simulink model "Quadrotor_Controller"  (R2019a)
settings: Solver=ode14x  StartTime=0.0  StopTime=10  FixedStep=1/100  RelTol=1e-3  EnableMultiTasking=on
undefined symbols (not defined in the file): Ap, cd, dfod, DiscIntNeverNeededParam, ioKd, ioKi, ioKp, Kd, Kp, kt, L, Newton, Pitch_0, Raphson, rho, Roll_0, Rp, X, Y, Z
libraries: sm_lib x122, fl_ps_legacy_lib x41, fl_lib x28, nesl_utility x14, sharedtransform x12, simulink x5, Electrical_Library x4, Mechanical_Library x4
(part 2 of 5)

== system Quadrotor_Controller/Controller/FOPI- GNCC IRID ==
  note: gam=-0.9693;
      | Ts=0.01;
      | dfod=irid_fod(gam,Ts,5);
  note: FOPI GNCC IRID
  In1 : Inport
  Discrete Transfer Fcn : DiscreteTransferFcn  Numerator=[0.0101201839324044,-0.0228427827690589,0.0162967440497079,-0.00320636053105791,-0.000423005899049262,8.95094110425754e-05]  Denominator=[1,-3.37446144143197,4.28685637101180,-2.49589501448942,0.632511381183536,-0.0490106070515154]
  Fractional DD : Subsystem  Commented=through  mask{gam=0.9693, ww=[1e-4,1e4], n=6, kF1=on, kF=Oustaloup filter, Ts=0.01}
      mask prompts: gam "Derivative order gamma"; ww "Frequency range [wb,wh]"; n "Apprixmation order"; kF1 "Is a low-pass filter required?"; kF "Filter type"; Ts "Sampling period"
      mask init: same as Quadrotor_Controller/Controller/FOPD/Fractional DD
      mask TypeOptions kF: Oustaloup filter | Modified Oustaloup filter | Matsuda-Fujii filter
      mask Display: disp(str)
  Saturation1 : Saturate  Commented=through  UpperLimit=2e3  LowerLimit=-2e3
  Saturation2 : Saturate  Commented=through  UpperLimit=100  LowerLimit=-100
  Sum : Sum
  k_i : Gain  Gain=0.1631
  k_p : Gain  Gain=9.9498
  Out1 : Outport
  wires:
  Fractional DD/1(Out1) -> Discrete Transfer Fcn/1  "DD_out"
  k_i/1 -> Fractional DD/1(In1)  "DD_input"
  In1/1 -> Sum/1, k_i/1  "P"
  Sum/1 -> k_p/1
  k_p/1 -> Saturation1/1
  Saturation1/1 -> Out1/1
  Saturation2/1 -> Sum/2  "D"
  Discrete Transfer Fcn/1 -> Saturation2/1

== system Quadrotor_Controller/Controller/FOPID ==
  note: FOPID controller
  In1 : Inport
  Fractional DD : Subsystem  mask{gam=0, ww=[1e-4,1e4], n=6, kF1=on, kF=Oustaloup filter, Ts=0.01}
      mask prompts: gam "Derivative order gamma"; ww "Frequency range [wb,wh]"; n "Apprixmation order"; kF1 "Is a low-pass filter required?"; kF "Filter type"; Ts "Sampling period"
      mask init: same as Quadrotor_Controller/Controller/FOPD/Fractional DD
      mask TypeOptions kF: Oustaloup filter | Modified Oustaloup filter | Matsuda-Fujii filter
      mask Display: disp(str)
  Fractional DD1 : Subsystem  mask{gam=1.5, ww=[1e-4,1e4], n=6, kF1=on, kF=Oustaloup filter, Ts=0.01}
      mask prompts: gam "Derivative order gamma"; ww "Frequency range [wb,wh]"; n "Apprixmation order"; kF1 "Is a low-pass filter required?"; kF "Filter type"; Ts "Sampling period"
      mask init: same as Quadrotor_Controller/Controller/FOPD/Fractional DD
      mask TypeOptions kF: Oustaloup filter | Modified Oustaloup filter | Matsuda-Fujii filter
      mask Display: disp(str)
  Gain1 : Gain  Gain=0
  Gain2 : Gain  Gain=2.6
  Gain3 : Gain  Gain=1.631
  Saturation1 : Saturate  UpperLimit=2e3  LowerLimit=-2e3
  Saturation2 : Saturate  UpperLimit=100  LowerLimit=-100
  Saturation3 : Saturate  UpperLimit=100  LowerLimit=-100
  Sum : Sum  Inputs=+++
  Out1 : Outport
  wires:
  Fractional DD/1(Out1) -> Saturation2/1  "DD_out"
  Gain1/1 -> Fractional DD/1(In1)  "DD_input"
  In1/1 -> Gain2/1, Gain3/1, Gain1/1  "P"
  Sum/1 -> Saturation1/1
  Saturation1/1 -> Out1/1
  Saturation2/1 -> Sum/2  "D"
  Gain2/1 -> Sum/1  "DD_input"
  Gain3/1 -> Fractional DD1/1(In1)  "DD_input"
  Fractional DD1/1(Out1) -> Saturation3/1  "DD_out"
  Saturation3/1 -> Sum/3  "D"

== system Quadrotor_Controller/Controller/FOPID NPM IRID with correct plant ==
  note: FOPID controller
  In1 : Inport
  Discrete Transfer Fcn : DiscreteTransferFcn  Numerator=[1,-3.16336631308587,3.71959536925849,-1.96568707629962,0.436885459917815,-0.0273811687803932]  Denominator=[0.0935414346693485,-0.239486864955964,0.209356682991156,-0.0676440492684792,0.00352282535674651,0.000822432073709469]  SampleTime=0.01
  Discrete-Time Integrator : DiscreteIntegrator  SampleTime=0.01  ICPrevOutput=DiscIntNeverNeededParam  ICPrevScaledInput=DiscIntNeverNeededParam
  Saturation1 : Saturate  UpperLimit=2e3  LowerLimit=-2e3
  Saturation3 : Saturate  UpperLimit=100  LowerLimit=-100
  Sum : Sum  Inputs=++|
  k_d : Gain  Gain=0.9588
  k_p : Gain  Gain=2.6
  Out1 : Outport
  wires:
  In1/1 -> k_p/1, k_d/1  "P"
  Sum/1 -> Saturation1/1
  Saturation1/1 -> Out1/1
  k_p/1 -> Sum/1  "DD_input"
  k_d/1 -> Discrete-Time Integrator/1  "DD_input"
  Discrete Transfer Fcn/1 -> Saturation3/1  "DD_out"
  Saturation3/1 -> Sum/2  "D"
  Discrete-Time Integrator/1 -> Discrete Transfer Fcn/1

== system Quadrotor_Controller/Controller/FOPID NPM IRID with wrong plant ==
  note: FOPID controller
  In1 : Inport
  Discrete Transfer Fcn : DiscreteTransferFcn  Numerator=[1,-3.16336631308587,3.71959536925849,-1.96568707629962,0.436885459917815,-0.0273811687803932]  Denominator=[0.0935414346693485,-0.239486864955964,0.209356682991156,-0.0676440492684792,0.00352282535674651,0.000822432073709469]  SampleTime=0.01
  Discrete-Time Integrator : DiscreteIntegrator  SampleTime=0.01  ICPrevOutput=DiscIntNeverNeededParam  ICPrevScaledInput=DiscIntNeverNeededParam
  Gain2 : Gain  Gain=2.6
  Gain3 : Gain  Gain=1.631
  Saturation1 : Saturate  UpperLimit=2e3  LowerLimit=-2e3
  Saturation3 : Saturate  UpperLimit=100  LowerLimit=-100
  Sum : Sum  Inputs=+++
  Out1 : Outport
  wires:
  In1/1 -> Gain2/1, Gain3/1  "P"
  Sum/1 -> Saturation1/1
  Saturation1/1 -> Out1/1
  Gain2/1 -> Sum/1  "DD_input"
  Gain3/1 -> Discrete-Time Integrator/1  "DD_input"
  Discrete Transfer Fcn/1 -> Saturation3/1  "DD_out"
  Saturation3/1 -> Sum/3  "D"
  Discrete-Time Integrator/1 -> Discrete Transfer Fcn/1

== system Quadrotor_Controller/Controller/Tuned IOPID ==
  In1 : Inport
  Derivative : Derivative
  Discrete-Time Integrator : DiscreteIntegrator  SampleTime=-1  ICPrevOutput=DiscIntNeverNeededParam  ICPrevScaledInput=DiscIntNeverNeededParam
  Gain : Gain  Gain=ioKp
  Gain1 : Gain  Gain=ioKi
  Gain2 : Gain  Gain=ioKd
  Gain3 : Gain
  Saturation : Saturate  UpperLimit=10  LowerLimit=-10
  Sum : Sum  Inputs=+++
  Sum1 : Sum  Inputs=-+|
  Sum2 : Sum  Inputs=|++
  Out1 : Outport
  wires:
  Sum/1 -> Sum1/1, Saturation/1
  Sum1/1 -> Gain3/1
  In1/1 -> Gain2/1, Gain/1, Gain1/1
  Sum2/1 -> Discrete-Time Integrator/1
  Derivative/1 -> Sum/3
  Gain/1 -> Sum/1
  Discrete-Time Integrator/1 -> Sum/2
  Gain1/1 -> Sum2/1
  Gain3/1 -> Sum2/2
  Gain2/1 -> Derivative/1
  Saturation/1 -> Sum1/2, Out1/1

== system Quadrotor_Controller/Controller/Velocity Subsystem ==
  note: to change time constant
  note: speed static error reduced
  Altitude_Rate : Inport
  In2 : Inport  Port=2
  Abs1 : Abs
  Constant : Constant  Value=8
  Constant1 : Constant  Value=8
  Constant2 : Constant  Value=0.324786114614273
  Constant3 : Constant  Value=19.7366420228035
  Discrete-Time Integrator : DiscreteIntegrator  SampleTime=-1  ICPrevOutput=DiscIntNeverNeededParam  ICPrevScaledInput=DiscIntNeverNeededParam
  Gain1 : Gain
  PID ZVel : simulink/Continuous/PID Controller  Controller=PID  Form=Parallel  TimeDomain=Discrete-time  SampleTime=0.01  IntegratorMethod=Forward Euler  FilterMethod=Forward Euler  ControllerParametersSource=external  P=2  I=6  D=0.324786114614273  UseFilter=on  N=19.7366420228035  TunerSelectOption=Transfer Function Based (PID Tuner App)  InitialConditionSource=internal  InitialConditionForIntegrator=0  InitialConditionForFilter=0  DifferentiatorICPrevScaledInput=0  ExternalReset=none  TrackingMode=off  Kt=1  LimitOutput=on  UpperSaturationLimit=5  LowerSaturationLimit=-5  LinearizeAsGain=on  AntiWindupMode=back-calculation  Kb=1  POutMin=[]  POutMax=[]  IOutMin=[]  IOutMax=[]  DOutMin=[]  DOutMax=[]  NOutMin=[]  NOutMax=[]  SumOutMin=[]  SumOutMax=[]  SaturationOutMin=[]  SaturationOutMax=[]  PParamDataTypeStr=single  PParamMin=[]  PParamMax=[]  IParamDataTypeStr=single  IParamMin=[]  IParamMax=[]  DParamDataTypeStr=single  DParamMin=[]  DParamMax=[]  NParamMin=[]  NParamMax=[]  KbParamMin=[]  KbParamMax=[]  KtParamMin=[]  KtParamMax=[]  KbOutMin=[]  KbOutMax=[]  KtOutMin=[]  KtOutMax=[]  IntegratorOutMin=[]  IntegratorOutMax=[]  FilterOutMin=[]  FilterOutMax=[]  SumI1OutMin=[]  SumI1OutMax=[]  SumI2OutMin=[]  SumI2OutMax=[]  SumI3OutMin=[]  SumI3OutMax=[]  SumI4OutMin=[]  SumI4OutMax=[]  SumDOutMin=[]  SumDOutMax=[]  DifferentiatorOutMin=[]  DifferentiatorOutMax=[]  FilterDiffOutCoefMin=[]  FilterDiffOutCoefMax=[]  ReciprocalOutMin=[]  ReciprocalOutMax=[]  SumDenOutMin=[]  SumDenOutMax=[]  SumNumOutMin=[]  SumNumOutMax=[]  DivideOutMin=[]  DivideOutMax=[]  IntegratorContinuousStateAttributes=''  IntegratorStateMustResolveToSignalObject=off  IntegratorRTWStateStorageClass=Auto  FilterContinuousStateAttributes=''  FilterStateMustResolveToSignalObject=off  FilterRTWStateStorageClass=Auto  ParallelPVariant=ExternalParameters  IdealPVariant=Disabled  IVariant=ExternalParameters  DVariant=ExternalParameters  IntegratorVariant=Discrete  SatVariant=Enabled  AWVariant=BackCalculation  PCopyVariant=Disabled  TRVariant=Disabled  FdbkBlocksVariant=Forward  IdealPFdbkVariant=Disabled  SatFdbkVariant=Disabled  DerivativeFilterVariant=ForwardEulerFilter  NVariant=ExternalParameters  NCopyVariant=Disabled  FilterICVariant=InternalICsFilter  IntegratorICVariant=InternalICs  ExternalResetVariant=Disabled  TRSumVariant=Passthrough  SumFdbkVariant=Disabled  SumVariant=Sum_PID
  PID ZVel1 : simulink/Continuous/PID Controller  Commented=on  Controller=PID  Form=Parallel  TimeDomain=Discrete-time  SampleTime=0.01  IntegratorMethod=Forward Euler  FilterMethod=Forward Euler  ControllerParametersSource=internal  P=2  I=1  D=0.324786114614273  UseFilter=on  N=19.7366420228035  TunerSelectOption=Transfer Function Based (PID Tuner App)  InitialConditionSource=internal  InitialConditionForIntegrator=0  InitialConditionForFilter=0  DifferentiatorICPrevScaledInput=0  ExternalReset=none  TrackingMode=off  Kt=1  LimitOutput=on  UpperSaturationLimit=5  LowerSaturationLimit=-5  LinearizeAsGain=on  AntiWindupMode=back-calculation  Kb=1  POutMin=[]  POutMax=[]  IOutMin=[]  IOutMax=[]  DOutMin=[]  DOutMax=[]  NOutMin=[]  NOutMax=[]  SumOutMin=[]  SumOutMax=[]  SaturationOutMin=[]  SaturationOutMax=[]  PParamDataTypeStr=single  PParamMin=[]  PParamMax=[]  IParamDataTypeStr=single  IParamMin=[]  IParamMax=[]  DParamDataTypeStr=single  DParamMin=[]  DParamMax=[]  NParamMin=[]  NParamMax=[]  KbParamMin=[]  KbParamMax=[]  KtParamMin=[]  KtParamMax=[]  KbOutMin=[]  KbOutMax=[]  KtOutMin=[]  KtOutMax=[]  IntegratorOutMin=[]  IntegratorOutMax=[]  FilterOutMin=[]  FilterOutMax=[]  SumI1OutMin=[]  SumI1OutMax=[]  SumI2OutMin=[]  SumI2OutMax=[]  SumI3OutMin=[]  SumI3OutMax=[]  SumI4OutMin=[]  SumI4OutMax=[]  SumDOutMin=[]  SumDOutMax=[]  DifferentiatorOutMin=[]  DifferentiatorOutMax=[]  FilterDiffOutCoefMin=[]  FilterDiffOutCoefMax=[]  ReciprocalOutMin=[]  ReciprocalOutMax=[]  SumDenOutMin=[]  SumDenOutMax=[]  SumNumOutMin=[]  SumNumOutMax=[]  DivideOutMin=[]  DivideOutMax=[]  IntegratorContinuousStateAttributes=''  IntegratorStateMustResolveToSignalObject=off  IntegratorRTWStateStorageClass=Auto  FilterContinuousStateAttributes=''  FilterStateMustResolveToSignalObject=off  FilterRTWStateStorageClass=Auto  ParallelPVariant=InternalParameters  IdealPVariant=Disabled  IVariant=InternalParameters  DVariant=InternalParameters  IntegratorVariant=Discrete  SatVariant=Enabled  AWVariant=BackCalculation  PCopyVariant=Disabled  TRVariant=Disabled  FdbkBlocksVariant=Forward  IdealPFdbkVariant=Disabled  SatFdbkVariant=Disabled  DerivativeFilterVariant=ForwardEulerFilter  NVariant=InternalParameters  NCopyVariant=Disabled  FilterICVariant=InternalICsFilter  IntegratorICVariant=InternalICs  ExternalResetVariant=Disabled  TRSumVariant=Passthrough  SumFdbkVariant=Disabled  SumVariant=Sum_PID
  Rate Transition : RateTransition  OutPortSampleTime=0.01
  Sum5 : Sum  Inputs=-+|
  To Workspace1 : ToWorkspace  VariableName=VelITAE  SaveFormat=Timeseries  SampleTime=-1
  Command : Outport
  wires:
  Discrete-Time Integrator/1 -> To Workspace1/1  "ZVel_ITAE"
  Rate Transition/1 -> Sum5/2
  Constant1/1 -> PID ZVel/3
  In2/1 -> Rate Transition/1
  Constant2/1 -> PID ZVel/4
  Gain1/1 -> Command/1
  Constant3/1 -> PID ZVel/5
  Abs1/1 -> Discrete-Time Integrator/1
  Sum5/1 -> PID ZVel/1, Abs1/1  "ZVel_Err"
  PID ZVel/1 -> Gain1/1
  Constant/1 -> PID ZVel/2
  Altitude_Rate/1 -> Sum5/1

== system Quadrotor_Controller/External Force/Rotor1 ==
  Display : Display
  External Force  and Torque1 : sm_lib/Forces and Torques/External Force and Torque  ForceResolutionFrame=AttachedFrame  EnableForceX=off  EnableForceY=off  EnableForceZ=on  EnableForce=off  TorqueResolutionFrame=AttachedFrame  EnableTorqueX=off  EnableTorqueY=off  EnableTorqueZ=off  EnableTorque=off
  PS Constant : fl_lib/Physical Signals/Sources/PS Constant  constant=1
  PS Constant1 : fl_lib/Physical Signals/Sources/PS Constant  constant=2*pi*L
  PS Constant2 : fl_lib/Physical Signals/Sources/PS Constant  constant=P
  PS Divide : fl_ps_legacy_lib/Legacy Physical Signals/Functions/PS Divide
      settings: SourceProductName=Simscape  SourceProductBaseCode=SS
  PS Gain1 : fl_ps_legacy_lib/Legacy Physical Signals/Functions/PS Gain  gain=1
      settings: SourceProductName=Simscape
  PS Product : fl_ps_legacy_lib/Legacy Physical Signals/Functions/PS Product
      settings: SourceProductName=Simscape  SourceProductBaseCode=SS
  PS Product1 : fl_ps_legacy_lib/Legacy Physical Signals/Functions/PS Product
      settings: SourceProductName=Simscape  SourceProductBaseCode=SS
  PS Saturation : fl_ps_legacy_lib/Legacy Physical Signals/Nonlinear Operators/PS Saturation  Commented=on  upper_limit=-0.01  lower_limit=-inf
      settings: SourceProductName=Simscape  SourceProductBaseCode=SS
  PS Subtract : fl_ps_legacy_lib/Legacy Physical Signals/Functions/PS Subtract
      settings: SourceProductName=Simscape  SourceProductBaseCode=SS
  PS-Simulink Converter : nesl_utility/PS-Simulink Converter  PhysicalDomain=network_engine_domain  SubClassName=ps_output  LeftPortType=input  RightPortType=output  PseudoPeriodic=off  Frequencies=[]  Unit=1  AffineConversion=off
  Pitch1 : fl_ps_legacy_lib/Legacy Physical Signals/Functions/PS Gain  gain=kt*rho*Ap*Rp*Rp
      settings: SourceProductName=Simscape
  Pitch2 : fl_ps_legacy_lib/Legacy Physical Signals/Functions/PS Gain  gain=-50
      settings: SourceProductName=Simscape
  Omega_x_body : PMIOPort  Side=Left
  AlphaProp : PMIOPort  Port=2  Side=Left
  Thrust : PMIOPort  Port=3  Side=Right
  Prop Speed : PMIOPort  Port=4  Side=Right
  wires:
  PS-Simulink Converter/1 -> Display/1
  connections:
  Pitch2/RConn1 -- Prop Speed/RConn1 -- External Force  and Torque1/LConn1
  External Force  and Torque1/RConn1 -- Thrust/RConn1
  PS Gain1/LConn1 -- AlphaProp/RConn1
  PS Subtract/LConn1 -- PS Constant/RConn1
  PS Subtract/LConn2 -- PS Product/RConn1
  Pitch2/LConn1 -- PS Product1/RConn1
  PS Product1/LConn1 -- Pitch1/RConn1
  Pitch1/LConn1 -- PS Divide/RConn1
  PS Product/LConn2 -- Omega_x_body/RConn1
  PS Constant1/RConn1 -- PS Product/LConn1
  PS Product1/LConn2 -- PS Gain1/RConn1 -- PS-Simulink Converter/LConn1
  PS Constant2/RConn1 -- PS Divide/LConn2
  PS Subtract/RConn1 -- PS Divide/LConn1

== system Quadrotor_Controller/External Force/Rotor2 ==
  Display : Display
  External Force  and Torque2 : sm_lib/Forces and Torques/External Force and Torque  ForceResolutionFrame=AttachedFrame  EnableForceX=off  EnableForceY=off  EnableForceZ=on  EnableForce=off  TorqueResolutionFrame=AttachedFrame  EnableTorqueX=off  EnableTorqueY=off  EnableTorqueZ=off  EnableTorque=off
  PS Constant : fl_lib/Physical Signals/Sources/PS Constant  constant=1
  PS Constant1 : fl_lib/Physical Signals/Sources/PS Constant  constant=-2*pi*L
  PS Constant2 : fl_lib/Physical Signals/Sources/PS Constant  constant=P
  PS Divide : fl_ps_legacy_lib/Legacy Physical Signals/Functions/PS Divide
      settings: SourceProductName=Simscape  SourceProductBaseCode=SS
  PS Gain1 : fl_ps_legacy_lib/Legacy Physical Signals/Functions/PS Gain  gain=1
      settings: SourceProductName=Simscape
  PS Product : fl_ps_legacy_lib/Legacy Physical Signals/Functions/PS Product
      settings: SourceProductName=Simscape  SourceProductBaseCode=SS
  PS Product1 : fl_ps_legacy_lib/Legacy Physical Signals/Functions/PS Product
      settings: SourceProductName=Simscape  SourceProductBaseCode=SS
  PS Saturation : fl_ps_legacy_lib/Legacy Physical Signals/Nonlinear Operators/PS Saturation  Commented=on  upper_limit=inf  lower_limit=0.01
      settings: SourceProductName=Simscape  SourceProductBaseCode=SS
  PS Subtract : fl_ps_legacy_lib/Legacy Physical Signals/Functions/PS Subtract
      settings: SourceProductName=Simscape  SourceProductBaseCode=SS
  PS-Simulink Converter : nesl_utility/PS-Simulink Converter  PhysicalDomain=network_engine_domain  SubClassName=ps_output  LeftPortType=input  RightPortType=output  PseudoPeriodic=off  Frequencies=[]  Unit=1  AffineConversion=off
  Pitch1 : fl_ps_legacy_lib/Legacy Physical Signals/Functions/PS Gain  gain=kt*rho*Ap*Rp*Rp
      settings: SourceProductName=Simscape
  Pitch2 : fl_ps_legacy_lib/Legacy Physical Signals/Functions/PS Gain  gain=50
      settings: SourceProductName=Simscape
  Omega_x_body : PMIOPort  Side=Left
  AlphaProp : PMIOPort  Port=2  Side=Left
  Thrust1 : PMIOPort  Port=3  Side=Right
  Prop Speed : PMIOPort  Port=4  Side=Right
  wires:
  PS-Simulink Converter/1 -> Display/1
  connections:
  External Force  and Torque2/RConn1 -- Thrust1/RConn1
  Pitch2/RConn1 -- Prop Speed/RConn1 -- External Force  and Torque2/LConn1
  PS Gain1/LConn1 -- AlphaProp/RConn1
  PS Subtract/LConn1 -- PS Constant/RConn1
  PS Subtract/LConn2 -- PS Product/RConn1
  Pitch2/LConn1 -- PS Product1/RConn1
  PS Product1/LConn1 -- Pitch1/RConn1
  Pitch1/LConn1 -- PS Divide/RConn1
  PS Product/LConn2 -- Omega_x_body/RConn1
  PS Constant1/RConn1 -- PS Product/LConn1
  PS Gain1/RConn1 -- PS Product1/LConn2 -- PS-Simulink Converter/LConn1
  PS Constant2/RConn1 -- PS Divide/LConn2
  PS Subtract/RConn1 -- PS Divide/LConn1

== system Quadrotor_Controller/External Force/Rotor3 ==
  Display : Display
  External Force  and Torque3 : sm_lib/Forces and Torques/External Force and Torque  ForceResolutionFrame=AttachedFrame  EnableForceX=off  EnableForceY=off  EnableForceZ=on  EnableForce=off  TorqueResolutionFrame=AttachedFrame  EnableTorqueX=off  EnableTorqueY=off  EnableTorqueZ=off  EnableTorque=off
  PS Constant : fl_lib/Physical Signals/Sources/PS Constant  constant=1
  PS Constant1 : fl_lib/Physical Signals/Sources/PS Constant  constant=-2*pi*L
  PS Constant2 : fl_lib/Physical Signals/Sources/PS Constant  constant=P
  PS Divide : fl_ps_legacy_lib/Legacy Physical Signals/Functions/PS Divide
      settings: SourceProductName=Simscape  SourceProductBaseCode=SS
  PS Gain1 : fl_ps_legacy_lib/Legacy Physical Signals/Functions/PS Gain  gain=1
      settings: SourceProductName=Simscape
  PS Product : fl_ps_legacy_lib/Legacy Physical Signals/Functions/PS Product
      settings: SourceProductName=Simscape  SourceProductBaseCode=SS
  PS Product1 : fl_ps_legacy_lib/Legacy Physical Signals/Functions/PS Product
      settings: SourceProductName=Simscape  SourceProductBaseCode=SS
  PS Saturation : fl_ps_legacy_lib/Legacy Physical Signals/Nonlinear Operators/PS Saturation  Commented=on  upper_limit=inf  lower_limit=0.01
      settings: SourceProductName=Simscape  SourceProductBaseCode=SS
  PS Subtract : fl_ps_legacy_lib/Legacy Physical Signals/Functions/PS Subtract
      settings: SourceProductName=Simscape  SourceProductBaseCode=SS
  PS-Simulink Converter : nesl_utility/PS-Simulink Converter  PhysicalDomain=network_engine_domain  SubClassName=ps_output  LeftPortType=input  RightPortType=output  PseudoPeriodic=off  Frequencies=[]  Unit=1  AffineConversion=off
  Pitch1 : fl_ps_legacy_lib/Legacy Physical Signals/Functions/PS Gain  gain=kt*rho*Ap*Rp*Rp
      settings: SourceProductName=Simscape
  Pitch3 : fl_ps_legacy_lib/Legacy Physical Signals/Functions/PS Gain  gain=50
      settings: SourceProductName=Simscape
  Omega_x_body : PMIOPort  Side=Left
  AlphaProp : PMIOPort  Port=2  Side=Left
  Thrust : PMIOPort  Port=3  Side=Right
  Prop Speed : PMIOPort  Port=4  Side=Right
  wires:
  PS-Simulink Converter/1 -> Display/1
  connections:
  External Force  and Torque3/LConn1 -- Prop Speed/RConn1 -- Pitch3/RConn1
  External Force  and Torque3/RConn1 -- Thrust/RConn1
  PS Gain1/LConn1 -- AlphaProp/RConn1
  PS Subtract/LConn1 -- PS Constant/RConn1
  PS Subtract/LConn2 -- PS Product/RConn1
  Pitch3/LConn1 -- PS Product1/RConn1
  PS Product1/LConn1 -- Pitch1/RConn1
  Pitch1/LConn1 -- PS Divide/RConn1
  PS Product/LConn2 -- Omega_x_body/RConn1
  PS Constant1/RConn1 -- PS Product/LConn1
  PS Product1/LConn2 -- PS Gain1/RConn1 -- PS-Simulink Converter/LConn1
  PS Constant2/RConn1 -- PS Divide/LConn2
  PS Subtract/RConn1 -- PS Divide/LConn1

== system Quadrotor_Controller/External Force/Rotor4 ==
  External Force  and Torque4 : sm_lib/Forces and Torques/External Force and Torque  ForceResolutionFrame=AttachedFrame  EnableForceX=off  EnableForceY=off  EnableForceZ=on  EnableForce=off  TorqueResolutionFrame=AttachedFrame  EnableTorqueX=off  EnableTorqueY=off  EnableTorqueZ=off  EnableTorque=off
  PS Constant : fl_lib/Physical Signals/Sources/PS Constant  constant=1
  PS Constant1 : fl_lib/Physical Signals/Sources/PS Constant  constant=2*pi*L
  PS Constant2 : fl_lib/Physical Signals/Sources/PS Constant  constant=P
  PS Divide : fl_ps_legacy_lib/Legacy Physical Signals/Functions/PS Divide
      settings: SourceProductName=Simscape  SourceProductBaseCode=SS
  PS Gain1 : fl_ps_legacy_lib/Legacy Physical Signals/Functions/PS Gain  gain=1
      settings: SourceProductName=Simscape
  PS Product : fl_ps_legacy_lib/Legacy Physical Signals/Functions/PS Product
      settings: SourceProductName=Simscape  SourceProductBaseCode=SS
  PS Product1 : fl_ps_legacy_lib/Legacy Physical Signals/Functions/PS Product
      settings: SourceProductName=Simscape  SourceProductBaseCode=SS
  PS Subtract : fl_ps_legacy_lib/Legacy Physical Signals/Functions/PS Subtract
      settings: SourceProductName=Simscape  SourceProductBaseCode=SS
  Pitch1 : fl_ps_legacy_lib/Legacy Physical Signals/Functions/PS Gain  gain=kt*rho*Ap*Rp*Rp
      settings: SourceProductName=Simscape
  Pitch4 : fl_ps_legacy_lib/Legacy Physical Signals/Functions/PS Gain  gain=-50
      settings: SourceProductName=Simscape
  Omega_x_body : PMIOPort  Side=Left
  AlphaProp : PMIOPort  Port=2  Side=Left
  Thrust : PMIOPort  Port=3  Side=Right
  Prop Speed : PMIOPort  Port=4  Side=Right
  connections:
  Thrust/RConn1 -- External Force  and Torque4/RConn1
  Pitch4/RConn1 -- External Force  and Torque4/LConn1 -- Prop Speed/RConn1
  AlphaProp/RConn1 -- PS Gain1/LConn1
  PS Subtract/RConn1 -- PS Divide/LConn1
  PS Constant2/RConn1 -- PS Divide/LConn2
  PS Gain1/RConn1 -- PS Product1/LConn2
  PS Constant1/RConn1 -- PS Product/LConn1
  PS Product/LConn2 -- Omega_x_body/RConn1
  Pitch1/LConn1 -- PS Divide/RConn1
  PS Product1/LConn1 -- Pitch1/RConn1
  Pitch4/LConn1 -- PS Product1/RConn1
  PS Subtract/LConn2 -- PS Product/RConn1
  PS Subtract/LConn1 -- PS Constant/RConn1

== system Quadrotor_Controller/Ground Stop/FloorStop1 ==
  6-DOF Joint1 : sm_lib/Joints/6-DOF Joint  SenseConstraintForce=off  SenseConstraintForceX=off  SenseConstraintForceY=off  SenseConstraintForceZ=off  SenseConstraintTorque=off  SenseConstraintTorqueX=off  SenseConstraintTorqueY=off  SenseConstraintTorqueZ=off  SenseTotalForce=off  SenseTotalForceX=off  SenseTotalForceY=off  SenseTotalForceZ=off  SenseTotalTorque=off  SenseTotalTorqueX=off  SenseTotalTorqueY=off  SenseTotalTorqueZ=off  CompositeWrenchDir=FollowerOnBase  CompositeWrenchFrame=BaseFrame  PxEquilibriumPosition=0  PxEquilibriumPositionUnits=m  PxSpringStiffness=0  PxSpringStiffnessUnits=N/m  PxDampingCoefficient=0  PxDampingCoefficientUnits=N/(m/s)  PxTorqueActuationMode=NoTorque  PxMotionActuationMode=ComputedMotion  PxSensePosition=off  PxSenseVelocity=off  PxSenseAcceleration=off  PxSenseTorqueForce=off  PxSenseLowerLimitTorqueForce=off  PxSenseUpperLimitTorqueForce=off  PxLowerLimitSpecify=off  PxLowerLimitBound=-1  PxLowerLimitBoundUnits=m  PxLowerLimitStiffness=1e6  PxLowerLimitStiffnessUnits=N/m  PxLowerLimitDamping=1e3  PxLowerLimitDampingUnits=N/(m/s)  PxLowerLimitTransitionRegionWidth=1e-4  PxLowerLimitTransitionRegionWidthUnits=m  PxUpperLimitSpecify=off  PxUpperLimitBound=1  PxUpperLimitBoundUnits=m  PxUpperLimitStiffness=1e6  PxUpperLimitStiffnessUnits=N/m  PxUpperLimitDamping=1e3  PxUpperLimitDampingUnits=N/(m/s)  PxUpperLimitTransitionRegionWidth=1e-4  PxUpperLimitTransitionRegionWidthUnits=m  PxPositionTargetSpecify=off  PxPositionTargetPriority=High  PxPositionTargetValue=1  PxPositionTargetValueUnits=m  PxVelocityTargetSpecify=off  PxVelocityTargetPriority=High  PxVelocityTargetValue=1  PxVelocityTargetValueUnits=m/s  PyEquilibriumPosition=0  PyEquilibriumPositionUnits=m  PySpringStiffness=0  PySpringStiffnessUnits=N/m  PyDampingCoefficient=0  PyDampingCoefficientUnits=N/(m/s)  PyTorqueActuationMode=NoTorque  PyMotionActuationMode=ComputedMotion  PySensePosition=off  PySenseVelocity=off  PySenseAcceleration=off  PySenseTorqueForce=off  PySenseLowerLimitTorqueForce=off  PySenseUpperLimitTorqueForce=off  PyLowerLimitSpecify=off  PyLowerLimitBound=-1  PyLowerLimitBoundUnits=m  PyLowerLimitStiffness=1e6  PyLowerLimitStiffnessUnits=N/m  PyLowerLimitDamping=1e3  PyLowerLimitDampingUnits=N/(m/s)  PyLowerLimitTransitionRegionWidth=1e-4  PyLowerLimitTransitionRegionWidthUnits=m  PyUpperLimitSpecify=off  PyUpperLimitBound=1  PyUpperLimitBoundUnits=m  PyUpperLimitStiffness=1e6  PyUpperLimitStiffnessUnits=N/m  PyUpperLimitDamping=1e3  PyUpperLimitDampingUnits=N/(m/s)  PyUpperLimitTransitionRegionWidth=1e-4  PyUpperLimitTransitionRegionWidthUnits=m  PyPositionTargetSpecify=off  PyPositionTargetPriority=High  PyPositionTargetValue=0  PyPositionTargetValueUnits=m  PyVelocityTargetSpecify=off  PyVelocityTargetPriority=High  PyVelocityTargetValue=0  PyVelocityTargetValueUnits=m/s  PzEquilibriumPosition=0  PzEquilibriumPositionUnits=m  PzSpringStiffness=0  PzSpringStiffnessUnits=N/m  PzDampingCoefficient=0  PzDampingCoefficientUnits=N/(m/s)  PzTorqueActuationMode=InputTorque  PzMotionActuationMode=ComputedMotion  PzSensePosition=on  PzSenseVelocity=on  PzSenseAcceleration=off  PzSenseTorqueForce=off  PzSenseLowerLimitTorqueForce=off  PzSenseUpperLimitTorqueForce=off  PzLowerLimitSpecify=off  PzLowerLimitBound=-1  PzLowerLimitBoundUnits=m  PzLowerLimitStiffness=1e6  PzLowerLimitStiffnessUnits=N/m  PzLowerLimitDamping=1e3  PzLowerLimitDampingUnits=N/(m/s)  PzLowerLimitTransitionRegionWidth=1e-4  PzLowerLimitTransitionRegionWidthUnits=m  PzUpperLimitSpecify=off  PzUpperLimitBound=1  PzUpperLimitBoundUnits=m  PzUpperLimitStiffness=1e6  PzUpperLimitStiffnessUnits=N/m  PzUpperLimitDamping=1e3  PzUpperLimitDampingUnits=N/(m/s)  PzUpperLimitTransitionRegionWidth=1e-4  PzUpperLimitTransitionRegionWidthUnits=m  PzPositionTargetSpecify=off  PzPositionTargetPriority=High  PzPositionTargetValue=-0.1  PzPositionTargetValueUnits=m  PzVelocityTargetSpecify=off  PzVelocityTargetPriority=High  PzVelocityTargetValue=0  PzVelocityTargetValueUnits=m/s  SphDefPosRotationMethod=None  SphDefPosRotationAngleUnits=deg  SphDefPosRotationStandardAxis=+Z  SphDefPosRotationAngle=0  SphDefPosRotationArbitraryAxis=[0 0 1]  SphDefPosFollAlignAxisA=+X  SphDefPosBaseAlignAxisA=+Y  SphDefPosFollAlignAxisB=+Y  SphDefPosBaseAlignAxisB=+Z  SphDefPosRotationSequenceAxes=FollowerAxes  SphDefPosRotationSequence=XYX  SphDefPosRotationSequenceAngles=[0 0 0]  SphDefPosRotationSequenceAnglesUnits=deg  SphDefPosRotationMatrix=[1 0 0; 0 1 0; 0 0 1]  SphEqPosRotationMethod=None  SphEqPosRotationAngleUnits=deg  SphEqPosRotationStandardAxis=+Z  SphEqPosRotationAngle=0  SphEqPosRotationArbitraryAxis=[0 0 1]  SphEqPosFollAlignAxisA=+X  SphEqPosBaseAlignAxisA=+Y  SphEqPosFollAlignAxisB=+Y  SphEqPosBaseAlignAxisB=+Z  SphEqPosRotationSequenceAxes=FollowerAxes  SphEqPosRotationSequence=XYX  SphEqPosRotationSequenceAngles=[0 0 0]  SphEqPosRotationSequenceAnglesUnits=deg  SphEqPosRotationMatrix=[1 0 0; 0 1 0; 0 0 1]  SphSpringStiffness=0  SphSpringStiffnessUnits=N*m/deg  SphDampingCoefficient=0  SphDampingCoefficientUnits=N*m/(deg/s)  SphActuateTorqueX=off  SphActuateTorqueY=off  SphActuateTorqueZ=off  SphActuateTorque=off  SphTorqueActuationMode=NoTorque  SphMotionActuationMode=ComputedMotion  SphActuationFrame=BaseFrame  SphSensePosition=off  SphSenseVelocityX=off  SphSenseVelocityY=off  SphSenseVelocityZ=off  SphSenseVelocity=off  SphSenseAccelerationX=off  SphSenseAccelerationY=off  SphSenseAccelerationZ=off  SphSenseAcceleration=off  SphSenseTorqueX=off  SphSenseTorqueY=off  SphSenseTorqueZ=off  SphSenseTorqueForce=off  SphSenseLowerLimitTorqueMag=off  SphSenseUpperLimitTorqueMag=off  SphSensingFrame=BaseFrame  SphLowerLimitSpecify=off  SphLowerLimitBound=15  SphLowerLimitBoundUnits=deg  SphLowerLimitStiffness=1e4  SphLowerLimitStiffnessUnits=N*m/deg  SphLowerLimitDamping=10  SphLowerLimitDampingUnits=N*m/(deg/s)  SphLowerLimitTransitionRegionWidth=0.1  SphLowerLimitTransitionRegionWidthUnits=deg  SphUpperLimitSpecify=off  SphUpperLimitBound=45  SphUpperLimitBoundUnits=deg  SphUpperLimitStiffness=1e4  SphUpperLimitStiffnessUnits=N*m/deg  SphUpperLimitDamping=10  SphUpperLimitDampingUnits=N*m/(deg/s)  SphUpperLimitTransitionRegionWidth=0.1  SphUpperLimitTransitionRegionWidthUnits=deg  SphPositionTargetRotationMethod=StandardAxis  SphPositionTargetRotationAngleUnits=deg  SphPositionTargetRotationStandardAxis=+X  SphPositionTargetRotationAngle=10  SphPositionTargetRotationArbitraryAxis=[0 0 1]  SphPositionTargetFollAlignAxisA=+X  SphPositionTargetBaseAlignAxisA=+Y  SphPositionTargetFollAlignAxisB=+Y  SphPositionTargetBaseAlignAxisB=+Z  SphPositionTargetRotationSequenceAxes=FollowerAxes  SphPositionTargetRotationSequence=XYX  SphPositionTargetRotationSequenceAngles=[0 0 0]  SphPositionTargetRotationSequenceAnglesUnits=deg  SphPositionTargetRotationMatrix=[1 0 0; 0 1 0; 0 0 1]  SphPositionTargetSpecify=off  SphPositionTargetPriority=High  SphVelocityTargetValue=[0 100 0]  SphVelocityTargetValueUnits=deg/s  SphVelocityTargetSpecify=off  SphVelocityTargetPriority=High  SphVelocityTargetInFollowerFrame=on
  Mechanical Translational Reference1 : fl_lib/Mechanical/Translational Elements/Mechanical Translational Reference
  PS Gain3 : fl_ps_legacy_lib/Legacy Physical Signals/Functions/PS Gain  gain=1
      settings: SourceProductName=Simscape
  PS Gain4 : fl_ps_legacy_lib/Legacy Physical Signals/Functions/PS Gain  gain=1
      settings: SourceProductName=Simscape
  Translational Simscape Intf1 : Subsystem
  Translational Hard Stop1 : fl_lib/Mechanical/Translational Elements/Translational Hard Stop  upper_bnd=100 m  lower_bnd=0 m  stiff_up=1e6 N/m  stiff_low=Spring N/m  D_up=1500 N/(m/s)  D_low=Damp N/(m/s)  model=3  transition=0.1 mm  v_specify=off  v_priority=High  v=0 m/s  v_nominal_specify=off  v_nominal_unit=m/s  v_nominal_value=1  f_specify=off  f_priority=High  f=0 N  f_nominal_specify=off  f_nominal_unit=N  f_nominal_value=1  x_specify=on  x_priority=High  x=Alt m  x_nominal_specify=off  x_nominal_unit=m  x_nominal_value=1
  Conn1 : PMIOPort  Side=Right
  Conn2 : PMIOPort  Port=2  Side=Left
  connections:
  6-DOF Joint1/RConn1 -- Conn1/RConn1
  Translational Hard Stop1/RConn1 -- Mechanical Translational Reference1/LConn1 -- Translational Simscape Intf1/RConn2
  Conn2/RConn1 -- 6-DOF Joint1/LConn1
  PS Gain3/RConn1 -- Translational Simscape Intf1/LConn1
  Translational Hard Stop1/LConn1 -- Translational Simscape Intf1/LConn2
  PS Gain3/LConn1 -- 6-DOF Joint1/RConn3
  Translational Simscape Intf1/RConn1 -- PS Gain4/LConn1
  PS Gain4/RConn1 -- 6-DOF Joint1/LConn2

== system Quadrotor_Controller/Ground Stop/FloorStop2 ==
  6-DOF Joint1 : sm_lib/Joints/6-DOF Joint  SenseConstraintForce=off  SenseConstraintForceX=off  SenseConstraintForceY=off  SenseConstraintForceZ=off  SenseConstraintTorque=off  SenseConstraintTorqueX=off  SenseConstraintTorqueY=off  SenseConstraintTorqueZ=off  SenseTotalForce=off  SenseTotalForceX=off  SenseTotalForceY=off  SenseTotalForceZ=off  SenseTotalTorque=off  SenseTotalTorqueX=off  SenseTotalTorqueY=off  SenseTotalTorqueZ=off  CompositeWrenchDir=FollowerOnBase  CompositeWrenchFrame=BaseFrame  PxEquilibriumPosition=0  PxEquilibriumPositionUnits=m  PxSpringStiffness=0  PxSpringStiffnessUnits=N/m  PxDampingCoefficient=0  PxDampingCoefficientUnits=N/(m/s)  PxTorqueActuationMode=NoTorque  PxMotionActuationMode=ComputedMotion  PxSensePosition=off  PxSenseVelocity=off  PxSenseAcceleration=off  PxSenseTorqueForce=off  PxSenseLowerLimitTorqueForce=off  PxSenseUpperLimitTorqueForce=off  PxLowerLimitSpecify=off  PxLowerLimitBound=-1  PxLowerLimitBoundUnits=m  PxLowerLimitStiffness=1e6  PxLowerLimitStiffnessUnits=N/m  PxLowerLimitDamping=1e3  PxLowerLimitDampingUnits=N/(m/s)  PxLowerLimitTransitionRegionWidth=1e-4  PxLowerLimitTransitionRegionWidthUnits=m  PxUpperLimitSpecify=off  PxUpperLimitBound=1  PxUpperLimitBoundUnits=m  PxUpperLimitStiffness=1e6  PxUpperLimitStiffnessUnits=N/m  PxUpperLimitDamping=1e3  PxUpperLimitDampingUnits=N/(m/s)  PxUpperLimitTransitionRegionWidth=1e-4  PxUpperLimitTransitionRegionWidthUnits=m  PxPositionTargetSpecify=off  PxPositionTargetPriority=High  PxPositionTargetValue=1  PxPositionTargetValueUnits=m  PxVelocityTargetSpecify=off  PxVelocityTargetPriority=High  PxVelocityTargetValue=1  PxVelocityTargetValueUnits=m/s  PyEquilibriumPosition=0  PyEquilibriumPositionUnits=m  PySpringStiffness=0  PySpringStiffnessUnits=N/m  PyDampingCoefficient=0  PyDampingCoefficientUnits=N/(m/s)  PyTorqueActuationMode=NoTorque  PyMotionActuationMode=ComputedMotion  PySensePosition=off  PySenseVelocity=off  PySenseAcceleration=off  PySenseTorqueForce=off  PySenseLowerLimitTorqueForce=off  PySenseUpperLimitTorqueForce=off  PyLowerLimitSpecify=off  PyLowerLimitBound=-1  PyLowerLimitBoundUnits=m  PyLowerLimitStiffness=1e6  PyLowerLimitStiffnessUnits=N/m  PyLowerLimitDamping=1e3  PyLowerLimitDampingUnits=N/(m/s)  PyLowerLimitTransitionRegionWidth=1e-4  PyLowerLimitTransitionRegionWidthUnits=m  PyUpperLimitSpecify=off  PyUpperLimitBound=1  PyUpperLimitBoundUnits=m  PyUpperLimitStiffness=1e6  PyUpperLimitStiffnessUnits=N/m  PyUpperLimitDamping=1e3  PyUpperLimitDampingUnits=N/(m/s)  PyUpperLimitTransitionRegionWidth=1e-4  PyUpperLimitTransitionRegionWidthUnits=m  PyPositionTargetSpecify=off  PyPositionTargetPriority=High  PyPositionTargetValue=0  PyPositionTargetValueUnits=m  PyVelocityTargetSpecify=off  PyVelocityTargetPriority=High  PyVelocityTargetValue=0  PyVelocityTargetValueUnits=m/s  PzEquilibriumPosition=0  PzEquilibriumPositionUnits=m  PzSpringStiffness=0  PzSpringStiffnessUnits=N/m  PzDampingCoefficient=0  PzDampingCoefficientUnits=N/(m/s)  PzTorqueActuationMode=InputTorque  PzMotionActuationMode=ComputedMotion  PzSensePosition=on  PzSenseVelocity=on  PzSenseAcceleration=off  PzSenseTorqueForce=off  PzSenseLowerLimitTorqueForce=off  PzSenseUpperLimitTorqueForce=off  PzLowerLimitSpecify=off  PzLowerLimitBound=-1  PzLowerLimitBoundUnits=m  PzLowerLimitStiffness=1e6  PzLowerLimitStiffnessUnits=N/m  PzLowerLimitDamping=1e3  PzLowerLimitDampingUnits=N/(m/s)  PzLowerLimitTransitionRegionWidth=1e-4  PzLowerLimitTransitionRegionWidthUnits=m  PzUpperLimitSpecify=off  PzUpperLimitBound=1  PzUpperLimitBoundUnits=m  PzUpperLimitStiffness=1e6  PzUpperLimitStiffnessUnits=N/m  PzUpperLimitDamping=1e3  PzUpperLimitDampingUnits=N/(m/s)  PzUpperLimitTransitionRegionWidth=1e-4  PzUpperLimitTransitionRegionWidthUnits=m  PzPositionTargetSpecify=off  PzPositionTargetPriority=High  PzPositionTargetValue=-0.1  PzPositionTargetValueUnits=m  PzVelocityTargetSpecify=off  PzVelocityTargetPriority=High  PzVelocityTargetValue=0  PzVelocityTargetValueUnits=m/s  SphDefPosRotationMethod=None  SphDefPosRotationAngleUnits=deg  SphDefPosRotationStandardAxis=+Z  SphDefPosRotationAngle=0  SphDefPosRotationArbitraryAxis=[0 0 1]  SphDefPosFollAlignAxisA=+X  SphDefPosBaseAlignAxisA=+Y  SphDefPosFollAlignAxisB=+Y  SphDefPosBaseAlignAxisB=+Z  SphDefPosRotationSequenceAxes=FollowerAxes  SphDefPosRotationSequence=XYX  SphDefPosRotationSequenceAngles=[0 0 0]  SphDefPosRotationSequenceAnglesUnits=deg  SphDefPosRotationMatrix=[1 0 0; 0 1 0; 0 0 1]  SphEqPosRotationMethod=None  SphEqPosRotationAngleUnits=deg  SphEqPosRotationStandardAxis=+Z  SphEqPosRotationAngle=0  SphEqPosRotationArbitraryAxis=[0 0 1]  SphEqPosFollAlignAxisA=+X  SphEqPosBaseAlignAxisA=+Y  SphEqPosFollAlignAxisB=+Y  SphEqPosBaseAlignAxisB=+Z  SphEqPosRotationSequenceAxes=FollowerAxes  SphEqPosRotationSequence=XYX  SphEqPosRotationSequenceAngles=[0 0 0]  SphEqPosRotationSequenceAnglesUnits=deg  SphEqPosRotationMatrix=[1 0 0; 0 1 0; 0 0 1]  SphSpringStiffness=0  SphSpringStiffnessUnits=N*m/deg  SphDampingCoefficient=0  SphDampingCoefficientUnits=N*m/(deg/s)  SphActuateTorqueX=off  SphActuateTorqueY=off  SphActuateTorqueZ=off  SphActuateTorque=off  SphTorqueActuationMode=NoTorque  SphMotionActuationMode=ComputedMotion  SphActuationFrame=BaseFrame  SphSensePosition=off  SphSenseVelocityX=off  SphSenseVelocityY=off  SphSenseVelocityZ=off  SphSenseVelocity=off  SphSenseAccelerationX=off  SphSenseAccelerationY=off  SphSenseAccelerationZ=off  SphSenseAcceleration=off  SphSenseTorqueX=off  SphSenseTorqueY=off  SphSenseTorqueZ=off  SphSenseTorqueForce=off  SphSenseLowerLimitTorqueMag=off  SphSenseUpperLimitTorqueMag=off  SphSensingFrame=BaseFrame  SphLowerLimitSpecify=off  SphLowerLimitBound=15  SphLowerLimitBoundUnits=deg  SphLowerLimitStiffness=1e4  SphLowerLimitStiffnessUnits=N*m/deg  SphLowerLimitDamping=10  SphLowerLimitDampingUnits=N*m/(deg/s)  SphLowerLimitTransitionRegionWidth=0.1  SphLowerLimitTransitionRegionWidthUnits=deg  SphUpperLimitSpecify=off  SphUpperLimitBound=45  SphUpperLimitBoundUnits=deg  SphUpperLimitStiffness=1e4  SphUpperLimitStiffnessUnits=N*m/deg  SphUpperLimitDamping=10  SphUpperLimitDampingUnits=N*m/(deg/s)  SphUpperLimitTransitionRegionWidth=0.1  SphUpperLimitTransitionRegionWidthUnits=deg  SphPositionTargetRotationMethod=StandardAxis  SphPositionTargetRotationAngleUnits=deg  SphPositionTargetRotationStandardAxis=+Y  SphPositionTargetRotationAngle=10  SphPositionTargetRotationArbitraryAxis=[0 0 1]  SphPositionTargetFollAlignAxisA=+X  SphPositionTargetBaseAlignAxisA=+Y  SphPositionTargetFollAlignAxisB=+Y  SphPositionTargetBaseAlignAxisB=+Z  SphPositionTargetRotationSequenceAxes=FollowerAxes  SphPositionTargetRotationSequence=XYX  SphPositionTargetRotationSequenceAngles=[0 0 0]  SphPositionTargetRotationSequenceAnglesUnits=deg  SphPositionTargetRotationMatrix=[1 0 0; 0 1 0; 0 0 1]  SphPositionTargetSpecify=off  SphPositionTargetPriority=High  SphVelocityTargetValue=[0 100 0]  SphVelocityTargetValueUnits=deg/s  SphVelocityTargetSpecify=off  SphVelocityTargetPriority=High  SphVelocityTargetInFollowerFrame=on
  Mechanical Translational Reference1 : fl_lib/Mechanical/Translational Elements/Mechanical Translational Reference
  PS Gain3 : fl_ps_legacy_lib/Legacy Physical Signals/Functions/PS Gain  gain=1
      settings: SourceProductName=Simscape
  PS Gain4 : fl_ps_legacy_lib/Legacy Physical Signals/Functions/PS Gain  gain=1
      settings: SourceProductName=Simscape
  Translational Simscape Intf1 : Subsystem
  Translational Hard Stop1 : fl_lib/Mechanical/Translational Elements/Translational Hard Stop  upper_bnd=100 m  lower_bnd=0 m  stiff_up=1e6 N/m  stiff_low=Spring N/m  D_up=1500 N/(m/s)  D_low=Damp N/(m/s)  model=3  transition=0.1 mm  v_specify=off  v_priority=High  v=0 m/s  v_nominal_specify=off  v_nominal_unit=m/s  v_nominal_value=1  f_specify=off  f_priority=High  f=0 N  f_nominal_specify=off  f_nominal_unit=N  f_nominal_value=1  x_specify=on  x_priority=High  x=Alt m  x_nominal_specify=off  x_nominal_unit=m  x_nominal_value=1
  Conn1 : PMIOPort  Side=Right
  Conn2 : PMIOPort  Port=2  Side=Left
  connections:
  PS Gain4/RConn1 -- 6-DOF Joint1/LConn2
  Translational Simscape Intf1/RConn1 -- PS Gain4/LConn1
  PS Gain3/LConn1 -- 6-DOF Joint1/RConn3
  Translational Hard Stop1/LConn1 -- Translational Simscape Intf1/LConn2
  PS Gain3/RConn1 -- Translational Simscape Intf1/LConn1
  Conn2/RConn1 -- 6-DOF Joint1/LConn1
  Translational Simscape Intf1/RConn2 -- Mechanical Translational Reference1/LConn1 -- Translational Hard Stop1/RConn1
  6-DOF Joint1/RConn1 -- Conn1/RConn1

== system Quadrotor_Controller/Ground Stop/FloorStop3 ==
  6-DOF Joint1 : sm_lib/Joints/6-DOF Joint  SenseConstraintForce=off  SenseConstraintForceX=off  SenseConstraintForceY=off  SenseConstraintForceZ=off  SenseConstraintTorque=off  SenseConstraintTorqueX=off  SenseConstraintTorqueY=off  SenseConstraintTorqueZ=off  SenseTotalForce=off  SenseTotalForceX=off  SenseTotalForceY=off  SenseTotalForceZ=off  SenseTotalTorque=off  SenseTotalTorqueX=off  SenseTotalTorqueY=off  SenseTotalTorqueZ=off  CompositeWrenchDir=FollowerOnBase  CompositeWrenchFrame=BaseFrame  PxEquilibriumPosition=0  PxEquilibriumPositionUnits=m  PxSpringStiffness=0  PxSpringStiffnessUnits=N/m  PxDampingCoefficient=0  PxDampingCoefficientUnits=N/(m/s)  PxTorqueActuationMode=NoTorque  PxMotionActuationMode=ComputedMotion  PxSensePosition=off  PxSenseVelocity=off  PxSenseAcceleration=off  PxSenseTorqueForce=off  PxSenseLowerLimitTorqueForce=off  PxSenseUpperLimitTorqueForce=off  PxLowerLimitSpecify=off  PxLowerLimitBound=-1  PxLowerLimitBoundUnits=m  PxLowerLimitStiffness=1e6  PxLowerLimitStiffnessUnits=N/m  PxLowerLimitDamping=1e3  PxLowerLimitDampingUnits=N/(m/s)  PxLowerLimitTransitionRegionWidth=1e-4  PxLowerLimitTransitionRegionWidthUnits=m  PxUpperLimitSpecify=off  PxUpperLimitBound=1  PxUpperLimitBoundUnits=m  PxUpperLimitStiffness=1e6  PxUpperLimitStiffnessUnits=N/m  PxUpperLimitDamping=1e3  PxUpperLimitDampingUnits=N/(m/s)  PxUpperLimitTransitionRegionWidth=1e-4  PxUpperLimitTransitionRegionWidthUnits=m  PxPositionTargetSpecify=off  PxPositionTargetPriority=High  PxPositionTargetValue=1  PxPositionTargetValueUnits=m  PxVelocityTargetSpecify=off  PxVelocityTargetPriority=High  PxVelocityTargetValue=1  PxVelocityTargetValueUnits=m/s  PyEquilibriumPosition=0  PyEquilibriumPositionUnits=m  PySpringStiffness=0  PySpringStiffnessUnits=N/m  PyDampingCoefficient=0  PyDampingCoefficientUnits=N/(m/s)  PyTorqueActuationMode=NoTorque  PyMotionActuationMode=ComputedMotion  PySensePosition=off  PySenseVelocity=off  PySenseAcceleration=off  PySenseTorqueForce=off  PySenseLowerLimitTorqueForce=off  PySenseUpperLimitTorqueForce=off  PyLowerLimitSpecify=off  PyLowerLimitBound=-1  PyLowerLimitBoundUnits=m  PyLowerLimitStiffness=1e6  PyLowerLimitStiffnessUnits=N/m  PyLowerLimitDamping=1e3  PyLowerLimitDampingUnits=N/(m/s)  PyLowerLimitTransitionRegionWidth=1e-4  PyLowerLimitTransitionRegionWidthUnits=m  PyUpperLimitSpecify=off  PyUpperLimitBound=1  PyUpperLimitBoundUnits=m  PyUpperLimitStiffness=1e6  PyUpperLimitStiffnessUnits=N/m  PyUpperLimitDamping=1e3  PyUpperLimitDampingUnits=N/(m/s)  PyUpperLimitTransitionRegionWidth=1e-4  PyUpperLimitTransitionRegionWidthUnits=m  PyPositionTargetSpecify=off  PyPositionTargetPriority=High  PyPositionTargetValue=0  PyPositionTargetValueUnits=m  PyVelocityTargetSpecify=off  PyVelocityTargetPriority=High  PyVelocityTargetValue=0  PyVelocityTargetValueUnits=m/s  PzEquilibriumPosition=0  PzEquilibriumPositionUnits=m  PzSpringStiffness=0  PzSpringStiffnessUnits=N/m  PzDampingCoefficient=0  PzDampingCoefficientUnits=N/(m/s)  PzTorqueActuationMode=InputTorque  PzMotionActuationMode=ComputedMotion  PzSensePosition=on  PzSenseVelocity=on  PzSenseAcceleration=off  PzSenseTorqueForce=off  PzSenseLowerLimitTorqueForce=off  PzSenseUpperLimitTorqueForce=off  PzLowerLimitSpecify=off  PzLowerLimitBound=-1  PzLowerLimitBoundUnits=m  PzLowerLimitStiffness=1e6  PzLowerLimitStiffnessUnits=N/m  PzLowerLimitDamping=1e3  PzLowerLimitDampingUnits=N/(m/s)  PzLowerLimitTransitionRegionWidth=1e-4  PzLowerLimitTransitionRegionWidthUnits=m  PzUpperLimitSpecify=off  PzUpperLimitBound=1  PzUpperLimitBoundUnits=m  PzUpperLimitStiffness=1e6  PzUpperLimitStiffnessUnits=N/m  PzUpperLimitDamping=1e3  PzUpperLimitDampingUnits=N/(m/s)  PzUpperLimitTransitionRegionWidth=1e-4  PzUpperLimitTransitionRegionWidthUnits=m  PzPositionTargetSpecify=off  PzPositionTargetPriority=High  PzPositionTargetValue=-0.1  PzPositionTargetValueUnits=m  PzVelocityTargetSpecify=off  PzVelocityTargetPriority=High  PzVelocityTargetValue=0  PzVelocityTargetValueUnits=m/s  SphDefPosRotationMethod=None  SphDefPosRotationAngleUnits=deg  SphDefPosRotationStandardAxis=+Z  SphDefPosRotationAngle=0  SphDefPosRotationArbitraryAxis=[0 0 1]  SphDefPosFollAlignAxisA=+X  SphDefPosBaseAlignAxisA=+Y  SphDefPosFollAlignAxisB=+Y  SphDefPosBaseAlignAxisB=+Z  SphDefPosRotationSequenceAxes=FollowerAxes  SphDefPosRotationSequence=XYX  SphDefPosRotationSequenceAngles=[0 0 0]  SphDefPosRotationSequenceAnglesUnits=deg  SphDefPosRotationMatrix=[1 0 0; 0 1 0; 0 0 1]  SphEqPosRotationMethod=None  SphEqPosRotationAngleUnits=deg  SphEqPosRotationStandardAxis=+Z  SphEqPosRotationAngle=0  SphEqPosRotationArbitraryAxis=[0 0 1]  SphEqPosFollAlignAxisA=+X  SphEqPosBaseAlignAxisA=+Y  SphEqPosFollAlignAxisB=+Y  SphEqPosBaseAlignAxisB=+Z  SphEqPosRotationSequenceAxes=FollowerAxes  SphEqPosRotationSequence=XYX  SphEqPosRotationSequenceAngles=[0 0 0]  SphEqPosRotationSequenceAnglesUnits=deg  SphEqPosRotationMatrix=[1 0 0; 0 1 0; 0 0 1]  SphSpringStiffness=0  SphSpringStiffnessUnits=N*m/deg  SphDampingCoefficient=0  SphDampingCoefficientUnits=N*m/(deg/s)  SphActuateTorqueX=off  SphActuateTorqueY=off  SphActuateTorqueZ=off  SphActuateTorque=off  SphTorqueActuationMode=NoTorque  SphMotionActuationMode=ComputedMotion  SphActuationFrame=BaseFrame  SphSensePosition=off  SphSenseVelocityX=off  SphSenseVelocityY=off  SphSenseVelocityZ=off  SphSenseVelocity=off  SphSenseAccelerationX=off  SphSenseAccelerationY=off  SphSenseAccelerationZ=off  SphSenseAcceleration=off  SphSenseTorqueX=off  SphSenseTorqueY=off  SphSenseTorqueZ=off  SphSenseTorqueForce=off  SphSenseLowerLimitTorqueMag=off  SphSenseUpperLimitTorqueMag=off  SphSensingFrame=BaseFrame  SphLowerLimitSpecify=off  SphLowerLimitBound=15  SphLowerLimitBoundUnits=deg  SphLowerLimitStiffness=1e4  SphLowerLimitStiffnessUnits=N*m/deg  SphLowerLimitDamping=10  SphLowerLimitDampingUnits=N*m/(deg/s)  SphLowerLimitTransitionRegionWidth=0.1  SphLowerLimitTransitionRegionWidthUnits=deg  SphUpperLimitSpecify=off  SphUpperLimitBound=45  SphUpperLimitBoundUnits=deg  SphUpperLimitStiffness=1e4  SphUpperLimitStiffnessUnits=N*m/deg  SphUpperLimitDamping=10  SphUpperLimitDampingUnits=N*m/(deg/s)  SphUpperLimitTransitionRegionWidth=0.1  SphUpperLimitTransitionRegionWidthUnits=deg  SphPositionTargetRotationMethod=StandardAxis  SphPositionTargetRotationAngleUnits=deg  SphPositionTargetRotationStandardAxis=+X  SphPositionTargetRotationAngle=10  SphPositionTargetRotationArbitraryAxis=[0 0 1]  SphPositionTargetFollAlignAxisA=+X  SphPositionTargetBaseAlignAxisA=+Y  SphPositionTargetFollAlignAxisB=+Y  SphPositionTargetBaseAlignAxisB=+Z  SphPositionTargetRotationSequenceAxes=FollowerAxes  SphPositionTargetRotationSequence=XYX  SphPositionTargetRotationSequenceAngles=[0 0 0]  SphPositionTargetRotationSequenceAnglesUnits=deg  SphPositionTargetRotationMatrix=[1 0 0; 0 1 0; 0 0 1]  SphPositionTargetSpecify=off  SphPositionTargetPriority=High  SphVelocityTargetValue=[0 100 0]  SphVelocityTargetValueUnits=deg/s  SphVelocityTargetSpecify=off  SphVelocityTargetPriority=High  SphVelocityTargetInFollowerFrame=on
  Mechanical Translational Reference1 : fl_lib/Mechanical/Translational Elements/Mechanical Translational Reference
  PS Gain3 : fl_ps_legacy_lib/Legacy Physical Signals/Functions/PS Gain  gain=1
      settings: SourceProductName=Simscape
  PS Gain4 : fl_ps_legacy_lib/Legacy Physical Signals/Functions/PS Gain  gain=1
      settings: SourceProductName=Simscape
  Translational Simscape Intf1 : Subsystem
  Translational Hard Stop1 : fl_lib/Mechanical/Translational Elements/Translational Hard Stop  upper_bnd=100 m  lower_bnd=0 m  stiff_up=1e6 N/m  stiff_low=Spring N/m  D_up=1500 N/(m/s)  D_low=Damp N/(m/s)  model=3  transition=0.1 mm  v_specify=off  v_priority=High  v=0 m/s  v_nominal_specify=off  v_nominal_unit=m/s  v_nominal_value=1  f_specify=off  f_priority=High  f=0 N  f_nominal_specify=off  f_nominal_unit=N  f_nominal_value=1  x_specify=on  x_priority=High  x=Alt m  x_nominal_specify=off  x_nominal_unit=m  x_nominal_value=1
  Conn1 : PMIOPort  Side=Right
  Conn2 : PMIOPort  Port=2  Side=Left
  connections:
  Translational Simscape Intf1/RConn1 -- PS Gain4/LConn1
  PS Gain3/LConn1 -- 6-DOF Joint1/RConn3
  Translational Hard Stop1/LConn1 -- Translational Simscape Intf1/LConn2
  PS Gain3/RConn1 -- Translational Simscape Intf1/LConn1
  Conn2/RConn1 -- 6-DOF Joint1/LConn1
  Translational Simscape Intf1/RConn2 -- Mechanical Translational Reference1/LConn1 -- Translational Hard Stop1/RConn1
  6-DOF Joint1/RConn1 -- Conn1/RConn1
  6-DOF Joint1/LConn2 -- PS Gain4/RConn1
